simulink model "sldemo_lct_bus"  (Simulink 7.6)
settings: Solver=ode5  StartTime=0.0  StopTime=30  RelTol=1e-3
PreLoadFcn:
  | load sldemo_lct_data.mat
libraries: simulink x1
Description:
  | Structure Arguments Using Buses
settings Model: Creator=The MathWorks Inc.  ExtModeAutoUpdateStatusClock=off
settings DataIOCC: SignalLoggingName=logsOut
settings OptimizationCC: InlineParams=on  InlineInvariantSignals=on  InitFltsAndDblsToZero=on  OptimizeModelRefInitCode=on  LifeSpan=1
settings DebuggingCC: CheckExecutionContextPreStartOutputMsg=on  CheckExecutionContextRuntimeOutputMsg=on  SignalResolutionControl=TryResolveAllWithWarning  SolverPrmCheckMsg=none  MultiTaskDSMMsg=warning  MultiTaskCondExecSysMsg=none  BusObjectLabelMismatch=error  StrictBusMsg=ErrorOnBusTreatedAsVector
settings HardwareCC: TargetHWDeviceType=32-bit Generic
settings ModelReferenceCC: UpdateModelReferenceTargets=IfOutOfDate
settings RTWCC: SystemTargetFile=ert.tlc  TemplateMakefile=ert_default_tmf  Description=Real-Time Workshop Embedded Coder (no auto configuration)  GenerateReport=on  RetainRTWFile=on  ProcessScript=ert_make_rtw_hook  CustomInclude=.\src  IncludeHyperlinkInReport=on  LaunchReport=on  IncludeERTFirstTime=on
settings CodeAppCC: IgnoreCustomStorageClasses=off
settings ERTTargetCC: TargetFcnLib=ansi_tfl_tmw.mat  MultiwordLength=2048  GenerateSampleERTMain=on  InlinedParameterPlacement=NonHierarchical  ERTCustomFileTemplate=example_file_process.tlc  ConvertIfToSwitch=off

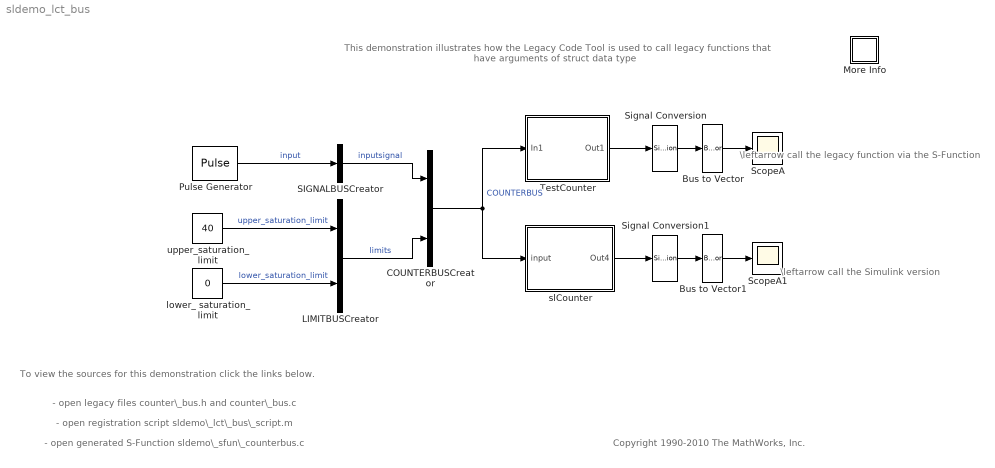
== system sldemo_lct_bus ==
  note: \leftarrow call the
      |     legacy function
      |      via the S-Function
  note: \leftarrow call the
      | Simulink version
  note: This demonstration illustrates how the Legacy Code Tool is used to
      | call legacy functions that have arguments of struct data type
  note: Copyright 1990-2010 The MathWorks, Inc.
  note: - open legacy files counter\_bus.h and counter\_bus.c
  note: To view the sources for this demonstration
      | click the links below.
  note: - open registration script sldemo\_lct\_bus\_script.m
  note: - open generated S-Function sldemo\_sfun\_counterbus.c
  Bus to Vector : BusToVector
  Bus to Vector1 : BusToVector
  COUNTERBUSCreator : BusCreator  Inputs=2  OutDataTypeStr=Bus: COUNTERBUS  NonVirtualBus=on
  LIMITBUSCreator : BusCreator  Inputs=2  OutDataTypeStr=Bus: LIMITBUS  NonVirtualBus=on
  More Info : Subsystem
      settings: OpenFcn=showdemo('sldemo_lct_bus_script')
      mask Display: disp('?')
  Pulse Generator : DiscretePulseGenerator  Amplitude=int32(1)  SampleTime=0.1
  SIGNALBUSCreator : BusCreator  Inputs=1  OutDataTypeStr=Bus: SIGNALBUS  NonVirtualBus=on
  ScopeA : Scope
      settings: TimeRange=30  YMax=50  SaveName=ScopeDataA  DataFormat=Array
  ScopeA1 : Scope
      settings: TimeRange=30  YMax=50  SaveName=ScopeDataA1  DataFormat=Array
  Signal Conversion : SignalConversion  ConversionOutput=Virtual bus
  Signal Conversion1 : SignalConversion  ConversionOutput=Virtual bus
  TestCounter : Subsystem
  lower_ saturation_ limit : Constant  Value=0  OutDataTypeStr=int32
  slCounter : Subsystem  TreatAsAtomicUnit=on
  upper_saturation_limit : Constant  Value=40  OutDataTypeStr=int32
  wires:
  upper_saturation_limit/1 -> LIMITBUSCreator/1  "upper_saturation_limit"
  lower_ saturation_ limit/1 -> LIMITBUSCreator/2  "lower_saturation_limit"
  LIMITBUSCreator/1 -> COUNTERBUSCreator/2  "limits"
  Pulse Generator/1 -> SIGNALBUSCreator/1  "input"
  SIGNALBUSCreator/1 -> COUNTERBUSCreator/1  "inputsignal"
  Signal Conversion/1 -> Bus to Vector/1
  TestCounter/1(Out1) -> Signal Conversion/1
  COUNTERBUSCreator/1 -> TestCounter/1(In1), slCounter/1(" input")  "COUNTERBUS"
  slCounter/1(Out4) -> Signal Conversion1/1
  Bus to Vector/1 -> ScopeA/1
  Signal Conversion1/1 -> Bus to Vector1/1
  Bus to Vector1/1 -> ScopeA1/1

== system sldemo_lct_bus/More Info ==

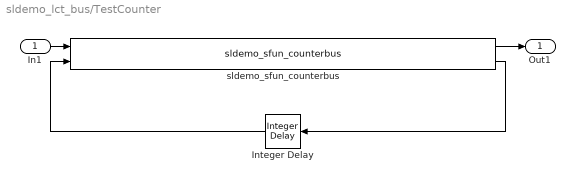
== system sldemo_lct_bus/TestCounter ==
  In1 : Inport  OutDataTypeStr=Bus: COUNTERBUS
  Integer Delay : simulink/Discrete/Integer Delay  vinit=0.0  samptime=-1  NumDelays=1
  sldemo_sfun_counterbus : S-Function  FunctionName=sldemo_sfun_counterbus  EnableBusSupport=off  mask(Legacy Function){SFunctionSpec=void counterbusFcn(COUNTERBUS u1[1], int32 u2, COUNTERBUS y1[1], int32 y2[1]), ShowSpec=on}
      mask prompts: ShowSpec "Display function specification"
      mask help:
      | This block allows you to call the legacy functions specified by the following Legacy Code Tool definition:
      | def.SFunctionName = 'sldemo_sfun_counterbus';
      | def.OutputFcnSpec = 'void counterbusFcn(COUNTERBUS u1[1], int32 u2, COUNTERBUS y1[1], int32 y2[1])';
      | def.HeaderFiles = {'counterbus.h'};
      | def.SourceFiles = {'counterbus.c'};
      | def.IncPaths = {'sldemo_lct_src'};
      | def.SrcPaths = {'sldemo_lct_src'};
      mask Help: <p>This block was generated automatically by the Legacy Code Tool. For detailed help on this tool, call<a href="matlab:legacy_code('help')"> legacy_code('help')</a>.</p>
      mask CallbackString:
      | |if strcmp(get_param(gcbh, 'ShowSpec'), 'on')
      |   set_param(gcbh, 'MaskDisplay', sprintf('fprintf(''%s'');', get_param(gcbh, 'SFunctionSpec')));
      | else
      |   set_param(gcbh, 'MaskDisplay', sprintf('fprintf(''%s'');', get_param(gcbh, 'FunctionName')));
      | end
      mask Display: fprintf('void counterbusFcn(COUNTERBUS u1[1], int32 u2, COUNTERBUS y1[1], int32 y2[1])');
  Out1 : Outport  OutDataTypeStr=Bus: COUNTERBUS
  wires:
  In1/1 -> sldemo_sfun_counterbus/1
  Integer Delay/1 -> sldemo_sfun_counterbus/2
  sldemo_sfun_counterbus/1 -> Out1/1
  sldemo_sfun_counterbus/2 -> Integer Delay/1

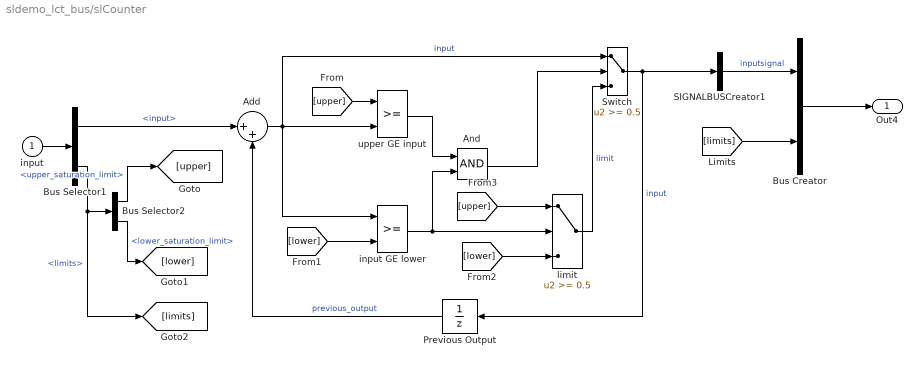
== system sldemo_lct_bus/slCounter ==
  " input" : Inport  OutDataTypeStr=Bus: COUNTERBUS
  " input GE lower" : RelationalOperator  Priority=1  InputSameDT=on
      settings: AttributesFormatString=\n
  " limit" : Switch  Threshold=0.5  SaturateOnIntegerOverflow=on  InputSameDT=on
  Add : Sum  Inputs=|++
  And : Logic
  Bus Creator : BusCreator  Inputs=2  OutDataTypeStr=Bus: COUNTERBUS  NonVirtualBus=on
  Bus Selector1 : BusSelector  OutputSignals=inputsignal.input,limits
  Bus Selector2 : BusSelector  OutputSignals=upper_saturation_limit,lower_saturation_limit
  Previous Output : UnitDelay  SampleTime=-1
  SIGNALBUSCreator1 : BusCreator  Inputs=1  OutDataTypeStr=Bus: SIGNALBUS  NonVirtualBus=on
  Switch : Switch  Threshold=0.5  SaturateOnIntegerOverflow=on  InputSameDT=on
  upper GE input : RelationalOperator  Priority=0  InputSameDT=on
      settings: AttributesFormatString=\n
  Out4 : Outport  OutDataTypeStr=Bus: COUNTERBUS
  wires:
  [upper] -> " limit"/1
  Switch/1 -> Previous Output/1, SIGNALBUSCreator1/1  "input"
  " limit"/1 -> Switch/3  "limit"
  upper GE input/1 -> And/1
  Previous Output/1 -> Add/2  "previous_output"
  [lower] -> " limit"/3
  [upper] -> upper GE input/1
  [lower] -> " input GE lower"/2
  " input GE lower"/1 -> And/2, " limit"/2
  And/1 -> Switch/2
  Add/1 -> " input GE lower"/1, upper GE input/2, Switch/1  "input"
  " input"/1 -> Bus Selector1/1
  Bus Selector1/2 -> Bus Selector2/1, [limits]  "<limits>"
  Bus Selector1/1 -> Add/1  "<input>"
  Bus Selector2/1 -> [upper]  "<upper_saturation_limit>"
  Bus Selector2/2 -> [lower]  "<lower_saturation_limit>"
  Bus Creator/1 -> Out4/1
  [limits] -> Bus Creator/2
  SIGNALBUSCreator1/1 -> Bus Creator/1  "inputsignal"
